simulink model "HalfAdder"  (R2023a)
settings: Solver=VariableStepAuto  StartTime=0.0  StopTime=1  RelTol=1e-3
settings Model: Creator=Admin  LastModifiedBy=Admin

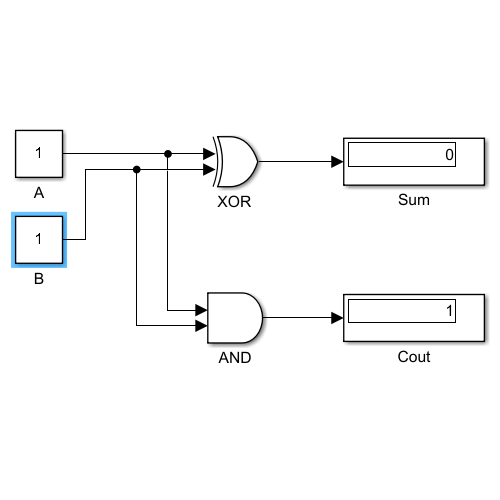
[thumbnail: Simulink's stored preview of the top-level diagram]
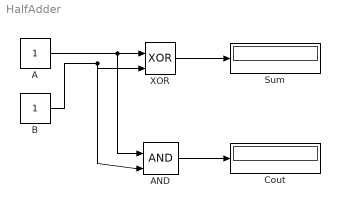
== system HalfAdder ==
  A : Constant
  AND : Logic  IconShape=distinctive  AllPortsSameDT=off  OutDataTypeStr=boolean
  B : Constant  SampleTime=-1
  Cout : Display
  Sum : Display
  XOR : Logic  Operator=XOR  IconShape=distinctive  AllPortsSameDT=off  OutDataTypeStr=boolean
  wires:
  A/1 -> AND/1, XOR/1
  B/1 -> AND/2, XOR/2
  XOR/1 -> Sum/1
  AND/1 -> Cout/1
